simulink model "Q2_Part_c"  (R2016b)
settings: Solver=VariableStepAuto  StartTime=0.0  StopTime=200  RelTol=1e-10  AbsTol=1e-10
libraries: cstblocks x2
settings Model: Creator=nadav  LastModifiedBy=nadav

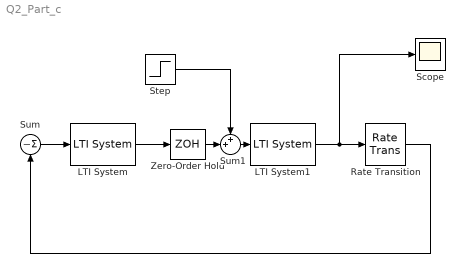
== system Q2_Part_c ==
  LTI System : cstblocks/LTI System  sys=Cd  IC=[]
  LTI System1 : cstblocks/LTI System  sys=P  IC=[]
  Rate Transition : RateTransition  OutPortSampleTime=ts
  Scope : Scope
  Step : Step  Time=0  SampleTime=0
  Sum : Sum  Inputs=||-
  Sum1 : Sum  Inputs=++|
  Zero-Order Hold : ZeroOrderHold  SampleTime=-1
  wires:
  LTI System/1 -> Zero-Order Hold/1
  LTI System1/1 -> Scope/1, Rate Transition/1
  Rate Transition/1 -> Sum/1
  Sum/1 -> LTI System/1
  Zero-Order Hold/1 -> Sum1/2
  Sum1/1 -> LTI System1/1
  Step/1 -> Sum1/1
